simulink model "Model_6DOF_2021a"  (R2021b)
settings: Solver=FixedStepAuto  StartTime=0.0  StopTime=Tfin  FixedStep=0.05  RelTol=1e-3
values from neighbouring files (symbols this model uses):
  adap = 1    [ctrl_mode_param.m]
  Ba_0 = [0 0 0 0 0 0]    [ctrl_mode_param.m]
  Bv_0 = [tgt_speed 0 0 0 0 0]    [ctrl_mode_param.m]
  Bx_0 = [0 0 tgt_depth 0 0 0]    [ctrl_mode_param.m]
  check_angle = 10    [ctrl_mode_param.m]
  Cp = [Cpx' ; Cpy' ; Cpz']    [ctrl_mode_param.m]
  Cp_prime = Cp*Dm    [ctrl_mode_param.m]
  ctrl_mode = 5    [run.m]
  dX_imposed = 10    [ctrl_mode_param.m]
  Seastate = 5    [ctrl_mode_param.m]    (also in run.m = 0)
  tgt_depth = -50    [ctrl_mode_param.m]
  tgt_pitch = 0    [ctrl_mode_param.m]
  tgt_speed = -5    [ctrl_mode_param.m]
  tgt_sway = 0    [ctrl_mode_param.m]
  tgt_yaw = 0    [ctrl_mode_param.m]
undefined symbols (not defined in the file or in its folder): Bb, dA_BP1, dA_BP2, dA_Hull, dA_PH, dA_Sail, dA_SProot, dA_X1a, dA_X1b, dA_X2a, dA_X2b, dA_X3a, dA_X3b, dA_X4a, dA_X4b, Ixx, Ixy, Ixz, Iyy, Iyz, Izz, Mb, n_BP1, n_BP2, n_Hull, n_PH, n_Sail, n_SProot, n_X2a, n_X2b, n_X3a, n_X4a, n_X4b, nt_BP1, nt_BP2, nt_Hull, nt_PH, nt_Sail, nt_SProot, nt_X1a, nt_X1b, nt_X2a, nt_X2b, nt_X3a, nt_X3b, nt_X4a, nt_X4b, vt1_BP1, vt1_BP2, vt1_Hull, vt1_PH, vt1_Sail, vt1_SProot, vt1_X1a, vt1_X1b, vt1_X2a, vt1_X2b, vt1_X3a, vt1_X3b, vt1_X4a ... (+36)
libraries: simulink x19
(part 4 of 6)

== system Model_6DOF_2021a/HDM/HDM B3/Wave, Virtual Mass and Hydrostatic/Wave Particle Motions/Hydrostatic Forces and Moments/X3 ==
  time : Inport
  Xearth : Inport  Port=2
  vert1 : Inport  Port=3
  vert2 : Inport  Port=4
  vert3 : Inport  Port=5
  dA : Inport  Port=6
  ntri : Inport  Port=7
  A_wave : Inport  Port=8
  k_wave : Inport  Port=9
  w_wave : Inport  Port=10
  rho : Inport  Port=11
  g : Inport  Port=12
  vert4 : Inport  Port=13
  vert5 : Inport  Port=14
  vert6 : Inport  Port=15
  dA1 : Inport  Port=16
  ntri1 : Inport  Port=17
  Zb : Inport  Port=18
  EAX : Inport  Port=19
  dX : Inport  Port=20
  Root_o : Inport  Port=21
  Add1 : Sum
  CG : Constant  Value=[32.3114; 0; 0;]
  MATLAB Function1 : MATLAB Function  TreatAsAtomicUnit=on
  MATLAB Function4 : MATLAB Function  TreatAsAtomicUnit=on
  Mux1 : Mux  Inputs=6
  Mux2 : Mux  Inputs=6
  Out1 : Outport
  wires:
  ntri1/1 -> MATLAB Function1/7(ntri)
  dA1/1 -> MATLAB Function1/6(dA)
  vert6/1 -> MATLAB Function1/5(vert3)
  vert5/1 -> MATLAB Function1/4(vert2)
  vert4/1 -> MATLAB Function1/3(vert1)
  Zb/1 -> MATLAB Function4/13(Zb), MATLAB Function1/13(Zb)
  vert2/1 -> MATLAB Function4/4(vert2)
  ntri/1 -> MATLAB Function4/7(ntri)
  time/1 -> MATLAB Function4/1(time), MATLAB Function1/1(time)
  vert1/1 -> MATLAB Function4/3(vert1)
  Mux1/1 -> Add1/2
  vert3/1 -> MATLAB Function4/5(vert3)
  Mux2/1 -> Add1/1
  MATLAB Function4/2(Fy_total) -> Mux2/2
  MATLAB Function4/6(Mz_total) -> Mux2/6
  g/1 -> MATLAB Function4/12(g), MATLAB Function1/12(g)
  k_wave/1 -> MATLAB Function4/9(k_wave), MATLAB Function1/9(k_wave)
  dA/1 -> MATLAB Function4/6(dA)
  MATLAB Function4/5(My_total) -> Mux2/5
  MATLAB Function1/3(Fz_total) -> Mux1/3
  Add1/1 -> Out1/1
  MATLAB Function1/1(Fx_total) -> Mux1/1
  MATLAB Function4/1(Fx_total) -> Mux2/1
  MATLAB Function1/4(Mx_total) -> Mux1/4
  A_wave/1 -> MATLAB Function4/8(A_wave), MATLAB Function1/8(A_wave)
  rho/1 -> MATLAB Function4/11(rho), MATLAB Function1/11(rho)
  Xearth/1 -> MATLAB Function4/2(Xearth), MATLAB Function1/2(Xearth)
  MATLAB Function1/2(Fy_total) -> Mux1/2
  w_wave/1 -> MATLAB Function4/10(w_wave), MATLAB Function1/10(w_wave)
  MATLAB Function4/4(Mx_total) -> Mux2/4
  MATLAB Function4/3(Fz_total) -> Mux2/3
  EAX/1 -> MATLAB Function4/14(EAX), MATLAB Function1/14(EAX)
  dX/1 -> MATLAB Function4/15(dX), MATLAB Function1/15(dX)
  Root_o/1 -> MATLAB Function4/16(origin), MATLAB Function1/16(origin)
  CG/1 -> MATLAB Function4/17(xcg), MATLAB Function1/17(xcg)
  MATLAB Function1/5(My_total) -> Mux1/5
  MATLAB Function1/6(Mz_total) -> Mux1/6

== system Model_6DOF_2021a/HDM/HDM B3/Wave, Virtual Mass and Hydrostatic/Wave Particle Motions/Hydrostatic Forces and Moments/X4 ==
  time : Inport
  Xearth : Inport  Port=2
  vert1 : Inport  Port=3
  vert2 : Inport  Port=4
  vert3 : Inport  Port=5
  dA : Inport  Port=6
  ntri : Inport  Port=7
  normal : Inport  Port=8
  A_wave : Inport  Port=9
  k_wave : Inport  Port=10
  w_wave : Inport  Port=11
  rho : Inport  Port=12
  g : Inport  Port=13
  vert4 : Inport  Port=14
  vert5 : Inport  Port=15
  vert6 : Inport  Port=16
  dA1 : Inport  Port=17
  ntri1 : Inport  Port=18
  Zb : Inport  Port=19
  EAX : Inport  Port=20
  dX : Inport  Port=21
  Root_o : Inport  Port=22
  Add1 : Sum
  CG : Constant  Value=[32.3114; 0; 0;]
  MATLAB Function1 : MATLAB Function  TreatAsAtomicUnit=on
  MATLAB Function4 : MATLAB Function  TreatAsAtomicUnit=on
  Mux1 : Mux  Inputs=6
  Mux2 : Mux  Inputs=6
  Out1 : Outport
  wires:
  MATLAB Function1/6(Mz_total) -> Mux1/6
  MATLAB Function1/5(My_total) -> Mux1/5
  CG/1 -> MATLAB Function1/17(xcg), MATLAB Function4/17(xcg)
  Root_o/1 -> MATLAB Function1/16(origin), MATLAB Function4/16(origin)
  dX/1 -> MATLAB Function1/15(dX), MATLAB Function4/15(dX)
  EAX/1 -> MATLAB Function1/14(EAX), MATLAB Function4/14(EAX)
  MATLAB Function4/3(Fz_total) -> Mux2/3
  MATLAB Function4/4(Mx_total) -> Mux2/4
  w_wave/1 -> MATLAB Function1/10(w_wave), MATLAB Function4/10(w_wave)
  MATLAB Function1/2(Fy_total) -> Mux1/2
  Xearth/1 -> MATLAB Function1/2(Xearth), MATLAB Function4/2(Xearth)
  rho/1 -> MATLAB Function4/11(rho), MATLAB Function1/11(rho)
  A_wave/1 -> MATLAB Function1/8(A_wave), MATLAB Function4/8(A_wave)
  MATLAB Function1/4(Mx_total) -> Mux1/4
  MATLAB Function4/1(Fx_total) -> Mux2/1
  MATLAB Function1/1(Fx_total) -> Mux1/1
  Add1/1 -> Out1/1
  MATLAB Function1/3(Fz_total) -> Mux1/3
  MATLAB Function4/5(My_total) -> Mux2/5
  dA/1 -> MATLAB Function4/6(dA)
  k_wave/1 -> MATLAB Function1/9(k_wave), MATLAB Function4/9(k_wave)
  g/1 -> MATLAB Function1/12(g), MATLAB Function4/12(g)
  MATLAB Function4/6(Mz_total) -> Mux2/6
  MATLAB Function4/2(Fy_total) -> Mux2/2
  Mux2/1 -> Add1/1
  vert3/1 -> MATLAB Function4/5(vert3)
  Mux1/1 -> Add1/2
  vert1/1 -> MATLAB Function4/3(vert1)
  time/1 -> MATLAB Function1/1(time), MATLAB Function4/1(time)
  normal/1 -> ?
  ntri/1 -> MATLAB Function4/7(ntri)
  vert2/1 -> MATLAB Function4/4(vert2)
  Zb/1 -> MATLAB Function1/13(Zb), MATLAB Function4/13(Zb)
  vert4/1 -> MATLAB Function1/3(vert1)
  vert5/1 -> MATLAB Function1/4(vert2)
  vert6/1 -> MATLAB Function1/5(vert3)
  dA1/1 -> MATLAB Function1/6(dA)
  ntri1/1 -> MATLAB Function1/7(ntri)

== system Model_6DOF_2021a/HDM/HDM B3/Wave, Virtual Mass and Hydrostatic/Wave Particle Motions/Hydrostatic Forces and Moments/XB ==
  time : Inport
  Xearth : Inport  Port=2
  vert1 : Inport  Port=3
  vert2 : Inport  Port=4
  vert3 : Inport  Port=5
  dA : Inport  Port=6
  ntri : Inport  Port=7
  normal : Inport  Port=8
  A_wave : Inport  Port=9
  k_wave : Inport  Port=10
  w_wave : Inport  Port=11
  rho : Inport  Port=12
  g : Inport  Port=13
  vert4 : Inport  Port=14
  vert5 : Inport  Port=15
  vert6 : Inport  Port=16
  dA1 : Inport  Port=17
  ntri1 : Inport  Port=18
  normal1 : Inport  Port=19
  Zb : Inport  Port=20
  EAX : Inport  Port=21
  dX : Inport  Port=22
  Root_o : Inport  Port=23
  Add1 : Sum
  CG : Constant  Value=[32.3114; 0; 0;]
  MATLAB Function1 : MATLAB Function  TreatAsAtomicUnit=on
  MATLAB Function4 : MATLAB Function  TreatAsAtomicUnit=on
  Mux1 : Mux  Inputs=6
  Mux2 : Mux  Inputs=6
  Out1 : Outport
  wires:
  MATLAB Function1/6(Mz_total) -> Mux1/6
  MATLAB Function1/5(My_total) -> Mux1/5
  CG/1 -> MATLAB Function1/17(xcg), MATLAB Function4/17(xcg)
  Root_o/1 -> MATLAB Function1/16(origin), MATLAB Function4/16(origin)
  dX/1 -> MATLAB Function1/15(dX), MATLAB Function4/15(dX)
  EAX/1 -> MATLAB Function1/14(EAX), MATLAB Function4/14(EAX)
  MATLAB Function4/3(Fz_total) -> Mux2/3
  MATLAB Function4/4(Mx_total) -> Mux2/4
  w_wave/1 -> MATLAB Function1/10(w_wave), MATLAB Function4/10(w_wave)
  MATLAB Function1/2(Fy_total) -> Mux1/2
  Xearth/1 -> MATLAB Function1/2(Xearth), MATLAB Function4/2(Xearth)
  rho/1 -> MATLAB Function1/11(rho), MATLAB Function4/11(rho)
  A_wave/1 -> MATLAB Function1/8(A_wave), MATLAB Function4/8(A_wave)
  MATLAB Function1/4(Mx_total) -> Mux1/4
  MATLAB Function4/1(Fx_total) -> Mux2/1
  MATLAB Function1/1(Fx_total) -> Mux1/1
  Add1/1 -> Out1/1
  MATLAB Function1/3(Fz_total) -> Mux1/3
  MATLAB Function4/5(My_total) -> Mux2/5
  dA/1 -> MATLAB Function4/6(dA)
  k_wave/1 -> MATLAB Function1/9(k_wave), MATLAB Function4/9(k_wave)
  g/1 -> MATLAB Function1/12(g), MATLAB Function4/12(g)
  MATLAB Function4/6(Mz_total) -> Mux2/6
  MATLAB Function4/2(Fy_total) -> Mux2/2
  Mux2/1 -> Add1/1
  vert3/1 -> MATLAB Function4/5(vert3)
  Mux1/1 -> Add1/2
  vert1/1 -> MATLAB Function4/3(vert1)
  time/1 -> MATLAB Function1/1(time), MATLAB Function4/1(time)
  normal/1 -> ?
  ntri/1 -> MATLAB Function4/7(ntri)
  vert2/1 -> MATLAB Function4/4(vert2)
  Zb/1 -> MATLAB Function1/13(Zb), MATLAB Function4/13(Zb)
  vert4/1 -> MATLAB Function1/3(vert1)
  vert5/1 -> MATLAB Function1/4(vert2)
  vert6/1 -> MATLAB Function1/5(vert3)
  dA1/1 -> MATLAB Function1/6(dA)
  ntri1/1 -> MATLAB Function1/7(ntri)
  normal1/1 -> ?

== matlab function Model_6DOF_2021a/Controller/HZZ/Subsystem/MATLAB Function ==
  data: rate input; dVrate output; trigger input; X5 input; dVprev input; dVmax input; dXmax input
function dVrate= fcn(rate,trigger,X5,dVprev,dVmax,dXmax)
if trigger == 0;
    dVrate=rate;
    zone=0
else
    if dVprev>0
       if dVprev>=dVmax
          if X5>=dXmax %dVprev
            dVrate=-rate;
            zone=2
          else
            dVrate=0;
            zone=3
          end
       elseif X5>=dXmax %dVprev
           dVrate=-rate;
           zone=4
       else
           zone=5
           dVrate=rate;
       end
    elseif dVprev<0
      if dVprev<=-dVmax
          if X5<=-dXmax%dVprev
            dVrate=rate;
            zone=-2
          else
            dVrate=0;
            zone=-3
          end
      elseif X5<=-dXmax%dVprev
          dVrate=rate;
          zone=-4
      else
          dVrate=-rate;
          zone=-5;
      end
    elseif dVprev==0
       if X5>0
           dVrate=rate
           zone=6
       else
           dVrate=-rate
           zone=-6
       end
    else
        zone=9
        dVrate=0;
    end
end

== matlab function Model_6DOF_2021a/Controller/PF+L1/pf_controller ==
  settings: updateMethod=DISCRETE
  data: Bv input; Bx input; dX output; ref input; n output; Cp parameter; Cp_prime parameter; stop output; adap input; pd output; NomegaNI output
function [dX,n,stop,pd,NomegaNI]   = fcn(Bv,Bx,ref,Cp,Cp_prime,adap)
%pd,NomegaNI,

%% Declare variables for integration and differentiation
Ts = 0.05; % Time step
stop = 0;
persistent gamma gammadot xuq xdq xur xdr RDT_prev RTI_prev ... 
    qerr_prev qerr_int_prev rerr_prev rerr_int_prev


%% Variables for feedback
x = Bx(1); y = Bx(2); z = Bx(3); phi = Bx(4); theta = Bx(5); psi = Bx(6);
p = [x;y;z];
uN = Bv(1); vN = Bv(2); wN = Bv(3); pB = Bv(4); qB=Bv(5); rB = Bv(6);
speed_cmd = ref;
uB = -uN; vB = -vN; wB = wN;

%% Control Parameters  
% Gains and parameters for PF
vcmd = 5; 
kgamma = 1; 
kR = 0.1; 
d = 250; 

% Gains for PF augmentation
Tsq = Ts; Tsr = Ts;
Amq = -0.1; Bmq = 0.25; Cmq = 0.4; 
Phiinvq = 50.1251; Lambdaq = 0.4;
Aoq = [-0.0496   -0.5024    0.5251; 1.3605   -0.5493    1.2008; -1.0756    0.8116   -1.5010]; 
Boq = [0.1240 ; -0.6198 ; 0.7748]; 
Coq = [0 0.8 0.64];
Amr = -0.1; Bmr = 0.25; Cmr = 0.4; 
Phiinvr = 50.1251; Lambdar = 0.4;
Aor = [-0.0300 -0.0192 -0.0082; 0.0156 0 0; 0 0.0078 0]; 
Bor = [0.25 ; 0 ; 0]; 
Cor = [0 0 0.1311];


% Autopilot Gain
KP_APq = 30*10^2;
KI_APq = 0*50*10^0;
KD_APq = 0;
KP_APr = 30*10^2;
KI_APr = 0*50*10^0;
KD_APr = 0;
% Speed controller gain
KP_n = 5;
FF_inv = 4;




%% Initialize
if isempty(gamma)
        gamma = 0; gammadot = 1;
        xuq = zeros(length(Aoq),1);
        xdq = Cmq'*inv(Cmq*Cmq')*qB;
        xur = zeros(length(Aor),1);
        xdr = Cmr'*inv(Cmr*Cmr')*rB;
        RDT_prev = zeros(3);
        RTI_prev = zeros(3);
        qerr_prev = 0;
        qerr_int_prev = 0;
        rerr_prev = 0;
        rerr_int_prev = 0;
        segment = 0;
end




%% Compute Rotation Matrices
alpha = -atan2(wB,sqrt(uB^2+vB^2));
beta = atan2(vB,uB);

RBW = [cos(alpha)*cos(beta) cos(alpha)*sin(beta) -sin(alpha);...
       -sin(beta)            cos(beta)             0;...
       cos(beta)*sin(alpha) sin(alpha)*sin(beta)  cos(alpha)];
   
RWB = RBW';


RNI = [ cos(psi)*cos(theta), cos(psi)*sin(phi)*sin(theta) - cos(phi)*sin(psi), sin(phi)*sin(psi) + cos(phi)*cos(psi)*sin(theta);
        cos(theta)*sin(psi), cos(phi)*cos(psi) + sin(phi)*sin(psi)*sin(theta), cos(phi)*sin(psi)*sin(theta) - cos(psi)*sin(phi);
         -sin(theta),                              cos(theta)*sin(phi),                              cos(phi)*cos(theta)];
     
RBN = [-1 0 0; 0 -1 0; 0 0 1];

RWI = RNI*RBN*RBW';

RWN = RBN*RWB;
RNW = RWN';


Tf = 5000;
pd = BernsteinPolyStable(Cp, gamma/Tf);
pd_prime = BernsteinPolyStable(Cp_prime, gamma/Tf);
pddot = pd_prime*gammadot;
if gamma >= Tf
    stop = 1;
end


t1hat = pd_prime/norm(pd_prime);
t2hat = [-pd_prime(2) ; pd_prime(1) ; 0 ]/norm([-pd_prime(2) ; pd_prime(1) ; 0 ]);
t3hat = cross(t1hat,t2hat);

RTI = [t1hat' ; t2hat' ; t3hat']';
RIT = RTI';







%% Compute gamma
gammadot = max(0.0001,((sqrt(uN^2+vN^2+wN^2)*RWI*[1;0;0] + kgamma*(p-pd))'*RTI*[1;0;0])/norm(pd_prime));
gamma = gamma + gammadot*Ts;







%% Compute desired angular rate
pT = RIT*(p-pd); %path following error

yT = pT(2); zT = pT(3);
toterr_y = yT; toterr_z = zT;
b1D = [d/(sqrt(d^2+toterr_y^2+toterr_z^2)) ; -toterr_y/(sqrt(d^2+toterr_y^2+toterr_z^2)) ; -toterr_z/(sqrt(d^2+toterr_y^2+toterr_z^2))];
b2D = [toterr_y/(sqrt(d^2+toterr_y^2)) ; d/(sqrt(d^2+toterr_y^2)) ; 0];
b3D = cross(b1D,b2D);
RDT = [b1D b2D b3D]; % Desired frame
% RTD = eye(3);
RTD = RDT';

Rtilde = RDT'*RIT*RWI;

eR = 0.5*[Rtilde(1,3); -Rtilde(1,2)];
PiR = [0 1 0 ; 0 0 1];


RDTdot = (RDT-RDT_prev)./Ts;
RTIdot = (RTI-RTI_prev)./Ts;

SDomegaDT = RTD*RDTdot;
DomegaDT = [-SDomegaDT(2,3); SDomegaDT(1,3) ; -SDomegaDT(1,2)];
STomegaTI = RIT*RTIdot;
TomegaTI = [-STomegaTI(2,3); STomegaTI(1,3) ; -STomegaTI(1,2)];

qc = [0 1 0]*Rtilde'*(RTD*TomegaTI + DomegaDT) - [1 0]*2*kR*eR;
rc = [0 0 1]*Rtilde'*(RTD*TomegaTI + DomegaDT) - [0 1]*2*kR*eR;


RNWdot = zeros(3,3);
SNomegaNW = RNW'*RNWdot;
NomegaNW = [-SNomegaNW(2,3) ; SNomegaNW(1,3); -SNomegaNW(1,2)];
NomegaNI = NomegaNW + RWN*[0;qc;rc];

q_ref = [0 1 0]*NomegaNI;
r_ref = [0 0 1]*NomegaNI;


RIW = RWI';
b1 = RWI(:,1);






%% L1 Augmentation - dive
ydq = Cmq*xdq;

sigmaq = -Phiinvq*expm(Lambdaq*(Amq/Lambdaq)*Tsq)*1*(ydq-qB);

xuq_next = expm(Aoq*Tsq)*xuq + inv(Aoq)*(expm(Aoq*Tsq)-eye(3))*(Boq*expm(-Amq*Tsq)*sigmaq);
Kgq = -inv(Cmq*inv(Amq)*Bmq);
udq = Kgq*q_ref - Coq*xuq;

xdq_next = expm(Amq*Tsq)*xdq + inv(Amq)*(expm(Amq*Tsq)-eye(length(Amq)))*(Bmq*udq + sigmaq);

qaug = udq;



%% Autopilot
if adap
    qerr = qaug - qB;
    %KI_APq = 0;
else
    qerr = q_ref - qB;
end
qerrint = qerr*Ts+qerr_int_prev;
qerrdot = (qerr-qerr_prev)/Ts;
dv = KP_APq*qerr+KI_APq*qerrint+KD_APq*qerrdot;


%% L1 Augmentation - steering
ydr = Cmr*xdr;

sigmar = -Phiinvr*expm(Lambdar*(Amr/Lambdar)*Tsr)*1*(ydr-rB);

xur_next = expm(Aor*Tsr)*xur + inv(Aor)*(expm(Aor*Tsr)-eye(3))*(Bor*expm(-Amr*Tsr)*sigmar);
Kgr = -inv(Cmr*inv(Amr)*Bmr);
udr = Kgr*r_ref - Cor*xur;

xdr_next = expm(Amr*Tsr)*xdr + inv(Amr)*(expm(Amr*Tsr)-eye(length(Amr)))*(Bmr*udr + sigmar);

raug = udr;




%% Autopilot
if adap
    rerr = raug - rB;
    %KI_APr = 0;
else
    rerr = r_ref - rB;
end
rerrint = rerr*Ts+rerr_int_prev;
rerrdot = (rerr-rerr_prev)/Ts;
dh = KP_APr*rerr+KI_APr*rerrint+KD_APr*rerrdot;



%% Control Allocation
d1 = -dv+dh; 
d2 = -dv-dh; 
d3 = dv-dh; 
d4 = dv+dh; 
d5 = dv; 

dX = [d1 ; d2 ; d3 ; d4 ; d5];






%% Speed Controller
% if x > -2500
%     s_d = ref;
% else
%     s_d = ref-.1/400*(x+2500);
% end
% n = -(s_d/FF_inv + KP_n*(s_d-uN));
%n = -(speed_cmd/FF_inv + KP_n*(speed_cmd-uN));

%speed_cmd = ref*min(1,.7*exp(-(gamma-400)/350)+.3);
n = -speed_cmd/FF_inv;



% gammaout = gamma;
% gammadotout = gammadot;
% pdes = pd;


%% Save variables for next loop
xuq = xuq_next;
xdq = xdq_next;
xur = xur_next;
xdr = xdr_next;
RDT_prev = RDT;
RTI_prev = RTI;
qerr_prev = qerr;
qerr_int_prev = qerrint;
rerr_prev = rerr;
rerr_int_prev = rerrint;


%% Functions requried for Bernstein Polynomials

function  poly_t  = BernsteinPoly(Cp,t,t0,tf)

% INPUTS:
% Cp is a matrix n by N+1 (n: dimension of polynomial, N: order of polynomial) 
% t is a time vector
% OUTPUT:
% poly_t: n-dimensional polynomial evaluated at each time t

% if t is a scalar, it returns the value of Bernstein Poly at t in [t0,tf]
% if t0 and tf are not provided, it returns the value of Bernstein Poly at t in [0,1]

% Written by: Venanzio Cichella       

%%%%%%%%%%%%%%%%%%%%%%%%%%%%%%%%%%%%%%%%%%%%%%



[~, N] = size(Cp);
N = N-1;

% if length(t) > 1
%     B = BernsteinMatrix_a2b(N,t)';
%     poly_t = Cp*B;
% else
%     if ~exist('t0','var')
%         B = BernsteinMatrix_a2b(N,t)';
%         poly_t = Cp*B;
%     else
%         B = BernsteinMatrix_a2b(N,t,t0,tf)';
%         poly_t = Cp*B;
%     end
% end
B = BernsteinMatrix_a2b(N,t,t0,tf)';
poly_t = Cp*B;






function  poly_t  = BernsteinPolyStable(Cp,t)

[m,n] = size(Cp);
poly_t = zeros(m,length(t));
count = 0;
for i = 1 : length(t)
    [~,poly_t(:,i)] = deCasteljau(Cp,t(i));
    count = count + 1;
end




function [Cpout, Pos] = deCasteljau(Cp,lambda)          
% Cpout are the control points of two curves.
% i.e.    cptsPA = Cpout(:, 1:length(Cp(1,:)));
%         cptsPB = Cpout(:, length(Cp(1,:)):end);
% Pos is the position at lambda
% lambda must be in [0,1]

[m,n] = size(Cp);
n = n-1;

A = (1-lambda)*eye(n,n);
B = lambda*eye(n,n);
C = zeros(n+1,n);

C(1:n,:) = C(1:n,:) + A; 
C(2:n+1,:) = C(2:n+1,:) + B;

Cpout = zeros(m,(n+1)+n);

Cptemp = Cp;
Cp1 = zeros(m,n);
Cp2 = zeros(m,n);

for i = n:-1:1
    Cptemp(:,1:i) = Cptemp(:,1:i+1)*C(1:i+1,1:i);
    Cp1(:,n+1-i) = Cptemp(:,1);
    Cp2(:,i) = Cptemp(:,i);
end

Cpout = [Cp(:,1) Cp1 Cp2(:,2:end) Cp(:,end)];
Pos = Cp1(:,end);





function b = BernsteinMatrix_a2b(N, t, tmin, tmax)

% Inputs: order N, time vector t = [t0 ... tm], no need for tmin and tmax.
% Output: b = [b0N(t0) b1N(t0) ... bNN(t0);
%              b0N(t1) b1N(t1) ... bNN(t1);
%              ...
%              b0N(tm) b1N(tm) ... bNN(tm);
% Use: If Cp is a row vector of N+1 control points,
%       the Nth order Bezier curve is given by xN=Cp*b';
% This function is used in BernsteinPoly

% Alternatively
% Inputs: order n, scalar time t', tmin and tmax
% Output: b = [b0n(t') b1n(t') ... bnn(t')]
% Use: If Cp is a row vector of N+1 control points,
%       the Nth order Bezier curve evaluated at t' is given by xn=Cp*b';
% Comment: This is more efficient but not as robust as de Casteljau
%           It works best for low-order curves

% Written by: Venanzio Cichella       

%%%%%%%%%%%%%%%%%%%%%%%%%%%%%%%%%%%%%%%%%%%%%%

if length(t) > 1
    tmax = t(length(t));
    tmin = t(1);
end

% if ~exist('tmin','var')
%     tmin = 0; tmax = 1;
% end



% compute B(j+1) = binomial(n, j), j = 0..n
t = t';
B = ones(N+1, 1); 
for j = 1:ceil(N/2)
  B(j+1) = B(j)*(N+1-j)/j;
  B(N+1-j) = B(j+1);
end
% compute T(i, j) = (t(i)-tmin)^j, TT(i, j) = (tmax-t(i))^(N-j)
T = ones(length(t), N+1);
TT = ones(length(t), N+1);
% turn a row t into a column t so that 
% we can do diag(t)*T(:,j) by t.*T(:,j)
tp = reshape(t, length(t), 1)-tmin;
ttp = tmax - t;
% Compute binomial(N, j)*(t(i)-tmin)^j*(tmax-t(i))^(N-j)
for j = 1:N 
  T(:, j+1) = tp .* T(:, j); 
  T(:, j) = T(:, j) .* B(j);
 TT(:,N+1-j) = ttp .* TT(:,N+2-j);
end

% Compute binomial(N, j)*(t(i)-tmin)^j*(tmax-t(i))^(N-j)/((tmax-tmin)^N)
b =  T.*TT./((tmax-tmin)^N);



function xN = LagrangePoly(x,tnodes,time)

%% Get polynomials
n = length(x);

basis_polynomials = cell(n,1); %basis polynomials for values t

for i = 1:n
    basis_polynomials{i} = 0;
    numerator = 1;
    denominator = 1;
    for k = 1:n
        if i~=k
            numerator = numerator.*(time-tnodes(k));
            denominator = denominator.*(tnodes(i)-tnodes(k));
        end
    end
    basis_polynomials{i} = numerator./denominator;
end


% then find the Lagrange polynomial coefficients
xN = 0;

for k = 1:n
    xN = xN + x(k)*basis_polynomials{k};
end

== matlab function Model_6DOF_2021a/Controller/VZZ/dV/MATLAB Function ==
  data: rate input; dVrate output; trigger input; X5 input; dVmax input; dXmax input; dVprev input
function dVrate = fcn(rate,trigger,X5,dVmax,dXmax,dVprev)
if trigger ==0;
    dVrate=rate;
    zone=0
else
    if dVprev>0
       if dVprev>=dVmax
          if X5>=dXmax %dVprev
            dVrate=-rate;
            zone=2
          else
            dVrate=0;
            zone=3
          end
       elseif X5>=dXmax %dVprev
           dVrate=-rate;
           zone=4
       else
           zone=5
           dVrate=rate;
       end
    elseif dVprev<0
      if dVprev<=-dVmax
          if X5<=-dXmax%dVprev
            dVrate=rate;
            zone=-2
          else
            dVrate=0;
            zone=-3
          end
      elseif X5<=-dXmax%dVprev
          dVrate=rate;
          zone=-4
      else
          dVrate=-rate;
          zone=-5;
      end
    elseif dVprev==0
       if X5>0
           dVrate=rate
           zone=6
       else
           dVrate=-rate
           zone=-6
       end
    else
        zone=9
        dVrate=0;
    end
end

== matlab function Model_6DOF_2021a/HDM/HDM B3/Wave, Virtual Mass and Hydrostatic/Wave Particle Motions/Hydrostatic Forces and Moments/XB/MATLAB Function1 ==
  data: time input; Xearth input; Fx_total output; vert1 input; vert2 input; vert3 input; dA input; ntri input; A_wave input; k_wave input; w_wave input; rho input; g input; Fy_total output; Fz_total output; Mx_total output; My_total output; Mz_total output; Zb input; EAX input; dX input; origin input; xcg input
function [Fx_total,Fy_total,Fz_total,Mx_total,My_total,Mz_total]= fcn(time,Xearth,vert1,vert2,vert3,dA,ntri,A_wave,k_wave,w_wave,rho,g,Zb,EAX,dX,origin,xcg)
%EAX=Appendage eulater angle in local coordinate
%its=number of time steps to skip writing grid

x_e=Xearth(1); y_e=Xearth(2); z_e=Xearth(3);
phi=Xearth(4); theta=Xearth(5); psi=Xearth(6);
phiX=EAX(1); thetaX=EAX(2); psiX=EAX(3);


RMat=[cos(theta)*cos(psi) -cos(phi)*sin(psi)+sin(phi)*sin(theta)*cos(psi)  sin(phi)*sin(psi)+cos(phi)*sin(theta)*cos(psi); ...
      cos(theta)*sin(psi)  cos(phi)*cos(psi)+sin(phi)*sin(theta)*sin(psi) -sin(phi)*cos(psi)+cos(phi)*sin(theta)*sin(psi); ...
     -sin(theta)                             sin(phi)*cos(theta)                             cos(phi)*cos(theta)];  
RMATX=[cos(thetaX)*cos(psiX) -cos(phiX)*sin(psiX)+sin(phiX)*sin(thetaX)*cos(psiX)  sin(phiX)*sin(psiX)+cos(phiX)*sin(thetaX)*cos(psiX); ...
      cos(thetaX)*sin(psiX)  cos(phiX)*cos(psiX)+sin(phiX)*sin(thetaX)*sin(psiX) -sin(phiX)*cos(psiX)+cos(phiX)*sin(thetaX)*sin(psiX); ...
     -sin(thetaX)                             sin(phiX)*cos(thetaX)                             cos(phiX)*cos(thetaX)];  
RMATD=[cos(0)*cos(dX) -cos(0)*sin(dX)+sin(0)*sin(0)*cos(dX)  sin(0)*sin(dX)+cos(0)*sin(0)*cos(dX); ...
      cos(0)*sin(dX)  cos(0)*cos(dX)+sin(0)*sin(0)*sin(dX) -sin(0)*cos(dX)+cos(0)*sin(0)*sin(dX); ...
     -sin(0)                             sin(0)*cos(0)                             cos(0)*cos(0)];  


%Rotating the vertices to put in ship coordinate
for i=1:ntri 
    V1=[vert1(i,1); vert1(i,2); vert1(i,3);];
    V2=[vert2(i,1); vert2(i,2); vert2(i,3);];
    V3=[vert3(i,1); vert3(i,2); vert3(i,3);];
        
    %rotating to local z coordinate
    V1_o=inv(RMATX)*(V1-origin*70.2+xcg);
    V2_o=inv(RMATX)*(V2-origin*70.2+xcg);
    V3_o=inv(RMATX)*(V3-origin*70.2+xcg);
    
    %rotating for corresponding appendage deflection
    V1_x=RMATD*V1_o;
    V2_x=RMATD*V2_o;
    V3_x=RMATD*V3_o;
    
        %re-positioning the appendage to local vectors
    V1_r=RMATX*V1_x;
    V2_r=RMATX*V2_x;
    V3_r=RMATX*V3_x;
    
    %re-assigning vertices
    
    for j=1:3
    vert1(i,j)=V1_r(j)+origin(j)*70.2-xcg(j);
    vert2(i,j)=V2_r(j)+origin(j)*70.2-xcg(j);
    vert3(i,j)=V3_r(j)+origin(j)*70.2-xcg(j);
    end  
end

 
%position of mid points in earth coordinate;
mp1=zeros(ntri,3);
mp2=zeros(ntri,3);
mp3=zeros(ntri,3);
nA =zeros(ntri,3);

P1=zeros(ntri,1);
P2=zeros(ntri,1);
P3=zeros(ntri,1);

%position vector of mid points from the CG
r1=zeros(ntri,3);
r2=zeros(ntri,3);
r3=zeros(ntri,3);

v1_w=zeros(ntri,3);
v2_w=zeros(ntri,3);
v3_w=zeros(ntri,3);
n_w=zeros(ntri,3);

%Area of triangle, product of area and unit normal, position vector to each mid-point

for i=1:ntri
    %Area of each triangle
    A=[vert2(i,1)-vert1(i,1); vert2(i,2)-vert1(i,2); vert2(i,3)-vert1(i,3);];
    B=[vert3(i,1)-vert1(i,1); vert3(i,2)-vert1(i,2); vert3(i,3)-vert1(i,3);];
    n=cross(A,B)/norm(cross(A,B));
    C=[n(1); n(2); n(3);];
    %C=[normal(i,1); normal(i,2); normal(i,3);];

    
    %A*n vector calculation
    for j=1:3
        nA(i,j)=dA(i).*C(j);    
    end
    
    %position vector to each mid point of each edge
    for j=1:3
        r1(i,j)=0.5*(vert1(i,j)+vert2(i,j));
        r2(i,j)=0.5*(vert1(i,j)+vert3(i,j));
        r3(i,j)=0.5*(vert2(i,j)+vert3(i,j));
    end
end

%computing mid point location between vertices in earth coordinate
for i=1:ntri
    MP1=RMat*[r1(i,1); r1(i,2); r1(i,3);]+[x_e; y_e; z_e;];
    MP2=RMat*[r2(i,1); r2(i,2); r2(i,3);]+[x_e; y_e; z_e;];
    MP3=RMat*[r3(i,1); r3(i,2); r3(i,3);]+[x_e; y_e; z_e;];
    
    v1i=RMat*[vert1(i,1); vert1(i,2); vert1(i,3);]+[x_e; y_e; z_e;];
    v2i=RMat*[vert2(i,1); vert2(i,2); vert2(i,3);]+[x_e; y_e; z_e;];
    v3i=RMat*[vert3(i,1); vert3(i,2); vert3(i,3);]+[x_e; y_e; z_e;];
    
    for j=1:3
        v1_w(i,j)=v1i(j); v2_w(i,j)=v2i(j); v3_w(i,j)=v3i(j);
        mp1(i,j)=MP1(j);  mp2(i,j)=MP2(j);  mp3(i,j)=MP3(j);
    end
end

for i=1:ntri
    A=[v2_w(i,1)-v1_w(i,1); v2_w(i,2)-v1_w(i,2); v2_w(i,3)-v1_w(i,3);];
    B=[v3_w(i,1)-v1_w(i,1); v3_w(i,2)-v1_w(i,2); v3_w(i,3)-v1_w(i,3);];
    n=cross(A,B)/norm(cross(A,B));
    dA(i,1)=0.5*norm(cross(A,B));
    n_w(i,1)=n(1); n_w(i,2)=n(2); n_w(i,3)=n(3);
end



%computing forces and moments for each triangle
Fx_total=0; Fy_total=0; Fz_total=0;
Mx_total=0; My_total=0; Mz_total=0;

for i=1:ntri
    p1=-rho*g*(mp1(i,3)-A_wave*exp(k_wave.*mp1(i,3)).*sin(k_wave*mp1(i,1)-w_wave.*time));
    p2=-rho*g*(mp2(i,3)-A_wave*exp(k_wave.*mp2(i,3)).*sin(k_wave*mp2(i,1)-w_wave.*time));
    p3=-rho*g*(mp3(i,3)-A_wave*exp(k_wave.*mp3(i,3)).*sin(k_wave*mp3(i,1)-w_wave.*time));
    
    dFx=-nA(i,1)*(p1+p2+p3)./3;
    dFy=-nA(i,2)*(p1+p2+p3)./3;
    dFz=-nA(i,3)*(p1+p2+p3)./3;
    
    dP =-p1.*[r1(i,1); r1(i,2); r1(i,3)-Zb;]...
        -p2.*[r2(i,1); r2(i,2); r2(i,3)-Zb;]...
        -p3.*[r3(i,1); r3(i,2); r3(i,3)-Zb;];
    N =[nA(i,1); nA(i,2); nA(i,3);];
    dM=cross(dP,N);
    Fx_total=Fx_total+dFx;
    Fy_total=Fy_total+dFy;
    Fz_total=Fz_total+dFz;
    Mx_total=Mx_total+dM(1)/3;
    My_total=My_total+dM(2)/3;
    Mz_total=Mz_total+dM(3)/3;
end
end

== matlab function Model_6DOF_2021a/HDM/Integration and Coord. Transfrom/Coordinate Transform/MATLAB Function2 ==
  data: Bx input; out output; Bv input
function out = fcn(Bx,Bv)
u = Bv(1); v = Bv(2); w = Bv(3); p = Bv(4); q = Bv(5); r = Bv(6);
x = Bx(1); y = Bx(2); z = Bx(3); phi = Bx(4); theta = Bx(5); psi = Bx(6);

Vx_ship=[u; v; w];
Vr_ship=[p; q; r];

RMat=[cos(theta)*cos(psi) -cos(phi)*sin(psi)+sin(phi)*sin(theta)*cos(psi)  sin(phi)*sin(psi)+cos(phi)*sin(theta)*cos(psi); ...
      cos(theta)*sin(psi)  cos(phi)*cos(psi)+sin(phi)*sin(theta)*sin(psi) -sin(phi)*cos(psi)+cos(phi)*sin(theta)*sin(psi); ...
              -sin(theta)                             sin(phi)*cos(theta)                             cos(phi)*cos(theta)];

QMat=[1  tan(theta)*sin(phi) tan(theta)*cos(phi); ...
      0  cos(phi)           -sin(phi); ...
      0  sin(phi)/cos(theta) cos(phi)/cos(theta)];
   
Vx_earth=RMat*Vx_ship;
Vr_earth=QMat*Vr_ship;


out = [Vx_earth(1); Vx_earth(2); Vx_earth(3); Vr_earth(1); Vr_earth(2); Vr_earth(3)];

== matlab function Model_6DOF_2021a/HDM/HDM B3/Wave, Virtual Mass and Hydrostatic/Wave Particle Motions/Hydrostatic Forces and Moments/X1/MATLAB Function1 ==
  data: time input; Xearth input; Fx_total output; vert1 input; vert2 input; vert3 input; dA input; ntri input; A_wave input; k_wave input; w_wave input; rho input; g input; Fy_total output; Fz_total output; Mx_total output; My_total output; Mz_total output; Zb input; EAX input; dX input; origin input; xcg input
function [Fx_total,Fy_total,Fz_total,Mx_total,My_total,Mz_total]= fcn(time,Xearth,vert1,vert2,vert3,dA,ntri,A_wave,k_wave,w_wave,rho,g,Zb,EAX,dX,origin,xcg)
%EAX=Appendage eulater angle in local coordinate
%its=number of time steps to skip writing grid
x_e=Xearth(1); y_e=Xearth(2); z_e=Xearth(3);
phi=Xearth(4); theta=Xearth(5); psi=Xearth(6);
phiX=EAX(1); thetaX=EAX(2); psiX=EAX(3);


RMat=[cos(theta)*cos(psi) -cos(phi)*sin(psi)+sin(phi)*sin(theta)*cos(psi)  sin(phi)*sin(psi)+cos(phi)*sin(theta)*cos(psi); ...
      cos(theta)*sin(psi)  cos(phi)*cos(psi)+sin(phi)*sin(theta)*sin(psi) -sin(phi)*cos(psi)+cos(phi)*sin(theta)*sin(psi); ...
     -sin(theta)                             sin(phi)*cos(theta)                             cos(phi)*cos(theta)];  
RMATX=[cos(thetaX)*cos(psiX) -cos(phiX)*sin(psiX)+sin(phiX)*sin(thetaX)*cos(psiX)  sin(phiX)*sin(psiX)+cos(phiX)*sin(thetaX)*cos(psiX); ...
      cos(thetaX)*sin(psiX)  cos(phiX)*cos(psiX)+sin(phiX)*sin(thetaX)*sin(psiX) -sin(phiX)*cos(psiX)+cos(phiX)*sin(thetaX)*sin(psiX); ...
     -sin(thetaX)                             sin(phiX)*cos(thetaX)                             cos(phiX)*cos(thetaX)];  
RMATD=[cos(0)*cos(dX) -cos(0)*sin(dX)+sin(0)*sin(0)*cos(dX)  sin(0)*sin(dX)+cos(0)*sin(0)*cos(dX); ...
      cos(0)*sin(dX)  cos(0)*cos(dX)+sin(0)*sin(0)*sin(dX) -sin(0)*cos(dX)+cos(0)*sin(0)*sin(dX); ...
     -sin(0)                             sin(0)*cos(0)                             cos(0)*cos(0)];  


%Rotating the vertices to put in ship coordinate
for i=1:ntri 
    V1=[vert1(i,1); vert1(i,2); vert1(i,3);];
    V2=[vert2(i,1); vert2(i,2); vert2(i,3);];
    V3=[vert3(i,1); vert3(i,2); vert3(i,3);];
        
    %rotating to local z coordinate
    V1_o=inv(RMATX)*(V1-origin*70.2+xcg);
    V2_o=inv(RMATX)*(V2-origin*70.2+xcg);
    V3_o=inv(RMATX)*(V3-origin*70.2+xcg);
    
    %rotating for corresponding appendage deflection
    V1_x=RMATD*V1_o;
    V2_x=RMATD*V2_o;
    V3_x=RMATD*V3_o;
    
        %re-positioning the appendage to local vectors
    V1_r=RMATX*V1_x;
    V2_r=RMATX*V2_x;
    V3_r=RMATX*V3_x;
    
    %re-assigning vertices
    
    for j=1:3
    vert1(i,j)=V1_r(j)+origin(j)*70.2-xcg(j);
    vert2(i,j)=V2_r(j)+origin(j)*70.2-xcg(j);
    vert3(i,j)=V3_r(j)+origin(j)*70.2-xcg(j);
    end  
end

 
%position of mid points in earth coordinate;
mp1=zeros(ntri,3);
mp2=zeros(ntri,3);
mp3=zeros(ntri,3);
nA =zeros(ntri,3);

P1=zeros(ntri,1);
P2=zeros(ntri,1);
P3=zeros(ntri,1);

%position vector of mid points from the CG
r1=zeros(ntri,3);
r2=zeros(ntri,3);
r3=zeros(ntri,3);

v1_w=zeros(ntri,3);
v2_w=zeros(ntri,3);
v3_w=zeros(ntri,3);
n_w=zeros(ntri,3);

%Area of triangle, product of area and unit normal, position vector to each mid-point

for i=1:ntri
    %Area of each triangle
    A=[vert2(i,1)-vert1(i,1); vert2(i,2)-vert1(i,2); vert2(i,3)-vert1(i,3);];
    B=[vert3(i,1)-vert1(i,1); vert3(i,2)-vert1(i,2); vert3(i,3)-vert1(i,3);];
    n=cross(A,B)/norm(cross(A,B));
    C=[n(1); n(2); n(3);];
    %C=[normal(i,1); normal(i,2); normal(i,3);];

    
    %A*n vector calculation
    for j=1:3
        nA(i,j)=dA(i).*C(j);    
    end
    
    %position vector to each mid point of each edge
    for j=1:3
        r1(i,j)=0.5*(vert1(i,j)+vert2(i,j));
        r2(i,j)=0.5*(vert1(i,j)+vert3(i,j));
        r3(i,j)=0.5*(vert2(i,j)+vert3(i,j));
    end
end

%computing mid point location between vertices in earth coordinate
for i=1:ntri
    MP1=RMat*[r1(i,1); r1(i,2); r1(i,3);]+[x_e; y_e; z_e;];
    MP2=RMat*[r2(i,1); r2(i,2); r2(i,3);]+[x_e; y_e; z_e;];
    MP3=RMat*[r3(i,1); r3(i,2); r3(i,3);]+[x_e; y_e; z_e;];
    
    v1i=RMat*[vert1(i,1); vert1(i,2); vert1(i,3);]+[x_e; y_e; z_e;];
    v2i=RMat*[vert2(i,1); vert2(i,2); vert2(i,3);]+[x_e; y_e; z_e;];
    v3i=RMat*[vert3(i,1); vert3(i,2); vert3(i,3);]+[x_e; y_e; z_e;];
    
    for j=1:3
        v1_w(i,j)=v1i(j); v2_w(i,j)=v2i(j); v3_w(i,j)=v3i(j);
        mp1(i,j)=MP1(j);  mp2(i,j)=MP2(j);  mp3(i,j)=MP3(j);
    end
end

for i=1:ntri
    A=[v2_w(i,1)-v1_w(i,1); v2_w(i,2)-v1_w(i,2); v2_w(i,3)-v1_w(i,3);];
    B=[v3_w(i,1)-v1_w(i,1); v3_w(i,2)-v1_w(i,2); v3_w(i,3)-v1_w(i,3);];
    n=cross(A,B)/norm(cross(A,B));
    dA(i,1)=0.5*norm(cross(A,B));
    n_w(i,1)=n(1); n_w(i,2)=n(2); n_w(i,3)=n(3);
end



%computing forces and moments for each triangle
Fx_total=0; Fy_total=0; Fz_total=0;
Mx_total=0; My_total=0; Mz_total=0;

for i=1:ntri
    p1=-rho*g*(mp1(i,3)-A_wave*exp(k_wave.*mp1(i,3)).*sin(k_wave*mp1(i,1)-w_wave.*time));
    p2=-rho*g*(mp2(i,3)-A_wave*exp(k_wave.*mp2(i,3)).*sin(k_wave*mp2(i,1)-w_wave.*time));
    p3=-rho*g*(mp3(i,3)-A_wave*exp(k_wave.*mp3(i,3)).*sin(k_wave*mp3(i,1)-w_wave.*time));
    
    dFx=-nA(i,1)*(p1+p2+p3)./3;
    dFy=-nA(i,2)*(p1+p2+p3)./3;
    dFz=-nA(i,3)*(p1+p2+p3)./3;
    
    dP =-p1.*[r1(i,1); r1(i,2); r1(i,3)-Zb;]...
        -p2.*[r2(i,1); r2(i,2); r2(i,3)-Zb;]...
        -p3.*[r3(i,1); r3(i,2); r3(i,3)-Zb;];
    N =[nA(i,1); nA(i,2); nA(i,3);];
    dM=cross(dP,N);
    Fx_total=Fx_total+dFx;
    Fy_total=Fy_total+dFy;
    Fz_total=Fz_total+dFz;
    Mx_total=Mx_total+dM(1)/3;
    My_total=My_total+dM(2)/3;
    Mz_total=Mz_total+dM(3)/3;
end
end

== matlab function Model_6DOF_2021a/HDM/HDM B3/Effective Veloicity Calclation/MATLAB Function ==
  data: nh input; n1 input; aX output; n2 input; n3 input; n4 input; nB input; urX1 input; urX2 input; urX3 input; urX4 input; urXB input; UeX output
function [aX,UeX] = fcn(nh,n1,n2,n3,n4,nB,urX1,urX2,urX3,urX4,urXB)

%urXi: relative velocity of rigid body motion and wave particle velocity to the ith stern plane
%ni  : base vector of i-th plane's axis direction
%nh  : base vector of the hull axis direction
IP=zeros(5,1); %IP determines the sign of the angle of attack. if the dot product is negative, angle is greater than 90degs.
aX=zeros(5,1);

np1=dot(nh,urX1)*nh+dot(n1,urX1)*n1;
np2=dot(nh,urX2)*nh+dot(n2,urX2)*n2;
np3=dot(nh,urX3)*nh+dot(n3,urX3)*n3;
np4=dot(nh,urX4)*nh+dot(n4,urX4)*n4;
npB=dot(nh,urXB)*nh+dot(nB,urXB)*nB;

arg1=dot(np1,urX1)/(norm(np1)*norm(urX1));
arg2=dot(np2,urX2)/(norm(np2)*norm(urX2));
arg3=dot(np3,urX3)/(norm(np3)*norm(urX3));
arg4=dot(np4,urX4)/(norm(np4)*norm(urX4));
arg5=dot(npB,urXB)/(norm(npB)*norm(urXB));

%to prevent numerical error: acos returns complex solution. used if statement
if arg1 >=1
   aX(1,1)=0;
else
   aX(1,1)=acos(arg1)*180/pi*sqrt(2);
end

if arg2 >=1
   aX(2,1)=0;
else
   aX(2,1)=acos(arg2)*180/pi*sqrt(2);
end

if arg3 >=1
   aX(3,1)=0;
else
   aX(3,1)=acos(arg3)*180/pi*sqrt(2);
end

if arg4 >=1
   aX(4,1)=0;
else
   aX(4,1)=acos(arg4)*180/pi*sqrt(2);
end

if arg5 >=1
   aX(5,1)=0;
else
   aX(5,1)=acos(arg5)*180/pi;
end

d1=cross(n1,nh);
d2=cross(n2,nh);
d3=cross(n3,nh);
d4=cross(n4,nh);
dB=cross(nB,nh);

IP(1,1)=dot(d1,urX1);
IP(2,1)=dot(d2,urX2);
IP(3,1)=dot(d3,urX3);
IP(4,1)=dot(d4,urX4);
IP(5,1)=dot(dB,urXB);

for i=1:5
    if IP(i,1)<0
        aX(i,1)=-aX(i,1)
    end
end    

UeX=[norm(urX1); norm(urX2); norm(urX3); norm(urX4); norm(urXB);];
end

== matlab function Model_6DOF_2021a/HDM/HDM B3/Wave, Virtual Mass and Hydrostatic/Wave Particle Motions/Hydrostatic Forces and Moments/X1/MATLAB Function4 ==
  data: time input; Xearth input; Fx_total output; vert1 input; vert2 input; vert3 input; dA input; ntri input; A_wave input; k_wave input; w_wave input; rho input; g input; Fy_total output; Fz_total output; Mx_total output; My_total output; Mz_total output; Zb input; EAX input; dX input; origin input; xcg input
function [Fx_total,Fy_total,Fz_total,Mx_total,My_total,Mz_total]= fcn(time,Xearth,vert1,vert2,vert3,dA,ntri,A_wave,k_wave,w_wave,rho,g,Zb,EAX,dX,origin,xcg)
%EAX=Appendage eulater angle in local coordinate
%its=number of time steps to skip writing grid

x_e=Xearth(1); y_e=Xearth(2); z_e=Xearth(3);
phi=Xearth(4); theta=Xearth(5); psi=Xearth(6);
phiX=EAX(1); thetaX=EAX(2); psiX=EAX(3);


RMat=[cos(theta)*cos(psi) -cos(phi)*sin(psi)+sin(phi)*sin(theta)*cos(psi)  sin(phi)*sin(psi)+cos(phi)*sin(theta)*cos(psi); ...
      cos(theta)*sin(psi)  cos(phi)*cos(psi)+sin(phi)*sin(theta)*sin(psi) -sin(phi)*cos(psi)+cos(phi)*sin(theta)*sin(psi); ...
     -sin(theta)                             sin(phi)*cos(theta)                             cos(phi)*cos(theta)];  
RMATX=[cos(thetaX)*cos(psiX) -cos(phiX)*sin(psiX)+sin(phiX)*sin(thetaX)*cos(psiX)  sin(phiX)*sin(psiX)+cos(phiX)*sin(thetaX)*cos(psiX); ...
      cos(thetaX)*sin(psiX)  cos(phiX)*cos(psiX)+sin(phiX)*sin(thetaX)*sin(psiX) -sin(phiX)*cos(psiX)+cos(phiX)*sin(thetaX)*sin(psiX); ...
     -sin(thetaX)                             sin(phiX)*cos(thetaX)                             cos(phiX)*cos(thetaX)];  
RMATD=[cos(0)*cos(dX) -cos(0)*sin(dX)+sin(0)*sin(0)*cos(dX)  sin(0)*sin(dX)+cos(0)*sin(0)*cos(dX); ...
      cos(0)*sin(dX)  cos(0)*cos(dX)+sin(0)*sin(0)*sin(dX) -sin(0)*cos(dX)+cos(0)*sin(0)*sin(dX); ...
     -sin(0)                             sin(0)*cos(0)                             cos(0)*cos(0)];  


%Rotating the vertices to put in ship coordinate
for i=1:ntri 
    V1=[vert1(i,1); vert1(i,2); vert1(i,3);];
    V2=[vert2(i,1); vert2(i,2); vert2(i,3);];
    V3=[vert3(i,1); vert3(i,2); vert3(i,3);];
        
    %rotating to local z coordinate
    V1_o=inv(RMATX)*(V1-origin*70.2+xcg);
    V2_o=inv(RMATX)*(V2-origin*70.2+xcg);
    V3_o=inv(RMATX)*(V3-origin*70.2+xcg);
    
    %rotating for corresponding appendage deflection
    V1_x=RMATD*V1_o;
    V2_x=RMATD*V2_o;
    V3_x=RMATD*V3_o;
    
        %re-positioning the appendage to local vectors
    V1_r=RMATX*V1_x;
    V2_r=RMATX*V2_x;
    V3_r=RMATX*V3_x;
    
    %re-assigning vertices
    
    for j=1:3
    vert1(i,j)=V1_r(j)+origin(j)*70.2-xcg(j);
    vert2(i,j)=V2_r(j)+origin(j)*70.2-xcg(j);
    vert3(i,j)=V3_r(j)+origin(j)*70.2-xcg(j);
    end  
end

 
%position of mid points in earth coordinate;
mp1=zeros(ntri,3);
mp2=zeros(ntri,3);
mp3=zeros(ntri,3);
nA =zeros(ntri,3);

P1=zeros(ntri,1);
P2=zeros(ntri,1);
P3=zeros(ntri,1);

%position vector of mid points from the CG
r1=zeros(ntri,3);
r2=zeros(ntri,3);
r3=zeros(ntri,3);

v1_w=zeros(ntri,3);
v2_w=zeros(ntri,3);
v3_w=zeros(ntri,3);
n_w=zeros(ntri,3);

%Area of triangle, product of area and unit normal, position vector to each mid-point

for i=1:ntri
    %Area of each triangle
    A=[vert2(i,1)-vert1(i,1); vert2(i,2)-vert1(i,2); vert2(i,3)-vert1(i,3);];
    B=[vert3(i,1)-vert1(i,1); vert3(i,2)-vert1(i,2); vert3(i,3)-vert1(i,3);];
    n=cross(A,B)/norm(cross(A,B));
    C=[n(1); n(2); n(3);];
    %C=[normal(i,1); normal(i,2); normal(i,3);];

    
    %A*n vector calculation
    for j=1:3
        nA(i,j)=dA(i).*C(j);    
    end
    
    %position vector to each mid point of each edge
    for j=1:3
        r1(i,j)=0.5*(vert1(i,j)+vert2(i,j));
        r2(i,j)=0.5*(vert1(i,j)+vert3(i,j));
        r3(i,j)=0.5*(vert2(i,j)+vert3(i,j));
    end
end

%computing mid point location between vertices in earth coordinate
for i=1:ntri
    MP1=RMat*[r1(i,1); r1(i,2); r1(i,3);]+[x_e; y_e; z_e;];
    MP2=RMat*[r2(i,1); r2(i,2); r2(i,3);]+[x_e; y_e; z_e;];
    MP3=RMat*[r3(i,1); r3(i,2); r3(i,3);]+[x_e; y_e; z_e;];
    
    v1i=RMat*[vert1(i,1); vert1(i,2); vert1(i,3);]+[x_e; y_e; z_e;];
    v2i=RMat*[vert2(i,1); vert2(i,2); vert2(i,3);]+[x_e; y_e; z_e;];
    v3i=RMat*[vert3(i,1); vert3(i,2); vert3(i,3);]+[x_e; y_e; z_e;];
    
    for j=1:3
        v1_w(i,j)=v1i(j); v2_w(i,j)=v2i(j); v3_w(i,j)=v3i(j);
        mp1(i,j)=MP1(j);  mp2(i,j)=MP2(j);  mp3(i,j)=MP3(j);
    end
end

for i=1:ntri
    A=[v2_w(i,1)-v1_w(i,1); v2_w(i,2)-v1_w(i,2); v2_w(i,3)-v1_w(i,3);];
    B=[v3_w(i,1)-v1_w(i,1); v3_w(i,2)-v1_w(i,2); v3_w(i,3)-v1_w(i,3);];
    n=cross(A,B)/norm(cross(A,B));
    dA(i,1)=0.5*norm(cross(A,B));
    n_w(i,1)=n(1); n_w(i,2)=n(2); n_w(i,3)=n(3);
end



%computing forces and moments for each triangle
Fx_total=0; Fy_total=0; Fz_total=0;
Mx_total=0; My_total=0; Mz_total=0;

for i=1:ntri
    p1=-rho*g*(mp1(i,3)-A_wave*exp(k_wave.*mp1(i,3)).*sin(k_wave*mp1(i,1)-w_wave.*time));
    p2=-rho*g*(mp2(i,3)-A_wave*exp(k_wave.*mp2(i,3)).*sin(k_wave*mp2(i,1)-w_wave.*time));
    p3=-rho*g*(mp3(i,3)-A_wave*exp(k_wave.*mp3(i,3)).*sin(k_wave*mp3(i,1)-w_wave.*time));
    
    dFx=-nA(i,1)*(p1+p2+p3)./3;
    dFy=-nA(i,2)*(p1+p2+p3)./3;
    dFz=-nA(i,3)*(p1+p2+p3)./3;
    
    dP =-p1.*[r1(i,1); r1(i,2); r1(i,3)-Zb;]...
        -p2.*[r2(i,1); r2(i,2); r2(i,3)-Zb;]...
        -p3.*[r3(i,1); r3(i,2); r3(i,3)-Zb;];
    N =[nA(i,1); nA(i,2); nA(i,3);];
    dM=cross(dP,N);
    Fx_total=Fx_total+dFx;
    Fy_total=Fy_total+dFy;
    Fz_total=Fz_total+dFz;
    Mx_total=Mx_total+dM(1)/3;
    My_total=My_total+dM(2)/3;
    Mz_total=Mz_total+dM(3)/3;
end
end

== matlab function Model_6DOF_2021a/HDM/HDM B3/Wave, Virtual Mass and Hydrostatic/Wave Particle Motions/Hydrostatic Forces and Moments/X2/MATLAB Function1 ==
  data: time input; Xearth input; Fx_total output; vert1 input; vert2 input; vert3 input; dA input; ntri input; A_wave input; k_wave input; w_wave input; rho input; g input; Fy_total output; Fz_total output; Mx_total output; My_total output; Mz_total output; Zb input; EAX input; dX input; origin input; xcg input
function [Fx_total,Fy_total,Fz_total,Mx_total,My_total,Mz_total]= fcn(time,Xearth,vert1,vert2,vert3,dA,ntri,A_wave,k_wave,w_wave,rho,g,Zb,EAX,dX,origin,xcg)
%EAX=Appendage eulater angle in local coordinate
%its=number of time steps to skip writing grid

x_e=Xearth(1); y_e=Xearth(2); z_e=Xearth(3);
phi=Xearth(4); theta=Xearth(5); psi=Xearth(6);
phiX=EAX(1); thetaX=EAX(2); psiX=EAX(3);


RMat=[cos(theta)*cos(psi) -cos(phi)*sin(psi)+sin(phi)*sin(theta)*cos(psi)  sin(phi)*sin(psi)+cos(phi)*sin(theta)*cos(psi); ...
      cos(theta)*sin(psi)  cos(phi)*cos(psi)+sin(phi)*sin(theta)*sin(psi) -sin(phi)*cos(psi)+cos(phi)*sin(theta)*sin(psi); ...
     -sin(theta)                             sin(phi)*cos(theta)                             cos(phi)*cos(theta)];  
RMATX=[cos(thetaX)*cos(psiX) -cos(phiX)*sin(psiX)+sin(phiX)*sin(thetaX)*cos(psiX)  sin(phiX)*sin(psiX)+cos(phiX)*sin(thetaX)*cos(psiX); ...
      cos(thetaX)*sin(psiX)  cos(phiX)*cos(psiX)+sin(phiX)*sin(thetaX)*sin(psiX) -sin(phiX)*cos(psiX)+cos(phiX)*sin(thetaX)*sin(psiX); ...
     -sin(thetaX)                             sin(phiX)*cos(thetaX)                             cos(phiX)*cos(thetaX)];  
RMATD=[cos(0)*cos(dX) -cos(0)*sin(dX)+sin(0)*sin(0)*cos(dX)  sin(0)*sin(dX)+cos(0)*sin(0)*cos(dX); ...
      cos(0)*sin(dX)  cos(0)*cos(dX)+sin(0)*sin(0)*sin(dX) -sin(0)*cos(dX)+cos(0)*sin(0)*sin(dX); ...
     -sin(0)                             sin(0)*cos(0)                             cos(0)*cos(0)];  


%Rotating the vertices to put in ship coordinate
for i=1:ntri 
    V1=[vert1(i,1); vert1(i,2); vert1(i,3);];
    V2=[vert2(i,1); vert2(i,2); vert2(i,3);];
    V3=[vert3(i,1); vert3(i,2); vert3(i,3);];
        
    %rotating to local z coordinate
    V1_o=inv(RMATX)*(V1-origin*70.2+xcg);
    V2_o=inv(RMATX)*(V2-origin*70.2+xcg);
    V3_o=inv(RMATX)*(V3-origin*70.2+xcg);
    
    %rotating for corresponding appendage deflection
    V1_x=RMATD*V1_o;
    V2_x=RMATD*V2_o;
    V3_x=RMATD*V3_o;
    
        %re-positioning the appendage to local vectors
    V1_r=RMATX*V1_x;
    V2_r=RMATX*V2_x;
    V3_r=RMATX*V3_x;
    
    %re-assigning vertices
    
    for j=1:3
    vert1(i,j)=V1_r(j)+origin(j)*70.2-xcg(j);
    vert2(i,j)=V2_r(j)+origin(j)*70.2-xcg(j);
    vert3(i,j)=V3_r(j)+origin(j)*70.2-xcg(j);
    end  
end

 
%position of mid points in earth coordinate;
mp1=zeros(ntri,3);
mp2=zeros(ntri,3);
mp3=zeros(ntri,3);
nA =zeros(ntri,3);

P1=zeros(ntri,1);
P2=zeros(ntri,1);
P3=zeros(ntri,1);

%position vector of mid points from the CG
r1=zeros(ntri,3);
r2=zeros(ntri,3);
r3=zeros(ntri,3);

v1_w=zeros(ntri,3);
v2_w=zeros(ntri,3);
v3_w=zeros(ntri,3);
n_w=zeros(ntri,3);

%Area of triangle, product of area and unit normal, position vector to each mid-point

for i=1:ntri
    %Area of each triangle
    A=[vert2(i,1)-vert1(i,1); vert2(i,2)-vert1(i,2); vert2(i,3)-vert1(i,3);];
    B=[vert3(i,1)-vert1(i,1); vert3(i,2)-vert1(i,2); vert3(i,3)-vert1(i,3);];
    n=cross(A,B)/norm(cross(A,B));
    C=[n(1); n(2); n(3);];
    %C=[normal(i,1); normal(i,2); normal(i,3);];

    
    %A*n vector calculation
    for j=1:3
        nA(i,j)=dA(i).*C(j);    
    end
    
    %position vector to each mid point of each edge
    for j=1:3
        r1(i,j)=0.5*(vert1(i,j)+vert2(i,j));
        r2(i,j)=0.5*(vert1(i,j)+vert3(i,j));
        r3(i,j)=0.5*(vert2(i,j)+vert3(i,j));
    end
end

%computing mid point location between vertices in earth coordinate
for i=1:ntri
    MP1=RMat*[r1(i,1); r1(i,2); r1(i,3);]+[x_e; y_e; z_e;];
    MP2=RMat*[r2(i,1); r2(i,2); r2(i,3);]+[x_e; y_e; z_e;];
    MP3=RMat*[r3(i,1); r3(i,2); r3(i,3);]+[x_e; y_e; z_e;];
    
    v1i=RMat*[vert1(i,1); vert1(i,2); vert1(i,3);]+[x_e; y_e; z_e;];
    v2i=RMat*[vert2(i,1); vert2(i,2); vert2(i,3);]+[x_e; y_e; z_e;];
    v3i=RMat*[vert3(i,1); vert3(i,2); vert3(i,3);]+[x_e; y_e; z_e;];
    
    for j=1:3
        v1_w(i,j)=v1i(j); v2_w(i,j)=v2i(j); v3_w(i,j)=v3i(j);
        mp1(i,j)=MP1(j);  mp2(i,j)=MP2(j);  mp3(i,j)=MP3(j);
    end
end

for i=1:ntri
    A=[v2_w(i,1)-v1_w(i,1); v2_w(i,2)-v1_w(i,2); v2_w(i,3)-v1_w(i,3);];
    B=[v3_w(i,1)-v1_w(i,1); v3_w(i,2)-v1_w(i,2); v3_w(i,3)-v1_w(i,3);];
    n=cross(A,B)/norm(cross(A,B));
    dA(i,1)=0.5*norm(cross(A,B));
    n_w(i,1)=n(1); n_w(i,2)=n(2); n_w(i,3)=n(3);
end


%computing forces and moments for each triangle
Fx_total=0; Fy_total=0; Fz_total=0;
Mx_total=0; My_total=0; Mz_total=0;

for i=1:ntri
    p1=-rho*g*(mp1(i,3)-A_wave*exp(k_wave.*mp1(i,3)).*sin(k_wave*mp1(i,1)-w_wave.*time));
    p2=-rho*g*(mp2(i,3)-A_wave*exp(k_wave.*mp2(i,3)).*sin(k_wave*mp2(i,1)-w_wave.*time));
    p3=-rho*g*(mp3(i,3)-A_wave*exp(k_wave.*mp3(i,3)).*sin(k_wave*mp3(i,1)-w_wave.*time));
    
    dFx=-nA(i,1)*(p1+p2+p3)./3;
    dFy=-nA(i,2)*(p1+p2+p3)./3;
    dFz=-nA(i,3)*(p1+p2+p3)./3;
    
    dP =-p1.*[r1(i,1); r1(i,2); r1(i,3)-Zb;]...
        -p2.*[r2(i,1); r2(i,2); r2(i,3)-Zb;]...
        -p3.*[r3(i,1); r3(i,2); r3(i,3)-Zb;];
    N =[nA(i,1); nA(i,2); nA(i,3);];
    dM=cross(dP,N);
    Fx_total=Fx_total+dFx;
    Fy_total=Fy_total+dFy;
    Fz_total=Fz_total+dFz;
    Mx_total=Mx_total+dM(1)/3;
    My_total=My_total+dM(2)/3;
    Mz_total=Mz_total+dM(3)/3;
end
end
